simulink model "Simulasi_DIY"  (R2024b)
settings: Solver=VariableStepAuto  StartTime=0.0  StopTime=10.0  RelTol=1e-3
values from neighbouring files (symbols this model uses):
  d1 = l1/2    (= 0.5)    [parameter.m]
  d2 = l2/2    (= 0.5)    [parameter.m]
  g = 9.81    [parameter.m]
  I1 = 1/12*m1*l1^2    (= 0.0833333333333)    [parameter.m]
  I2 = 1/12*m2*l2^2    (= 0.0833333333333)    [parameter.m]
  Kpx = 400    [parameter.m]
  Kpy = 400    [parameter.m]
  Kvx = 150    [parameter.m]
  Kvy = 150    [parameter.m]
  l1 = 1    [parameter.m]
  l2 = 1    [parameter.m]
  m1 = 1    [parameter.m]
  m2 = 1    [parameter.m]
  xt = -1    [main.m]    (also in parameter.m)
  yt = 1    [main.m]    (also in parameter.m)
undefined symbols (not defined in the file or in its folder): the_init
settings Model: Creator=WIN 10  LastModifiedBy=rifki
settings RTWCC: GPUComputeCapability=3.5

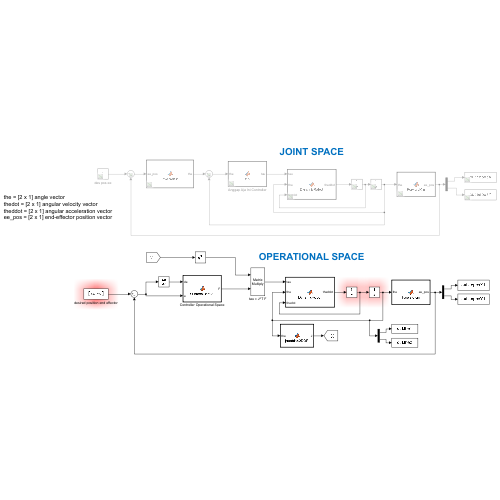
[thumbnail: Simulink's stored preview of the top-level diagram]
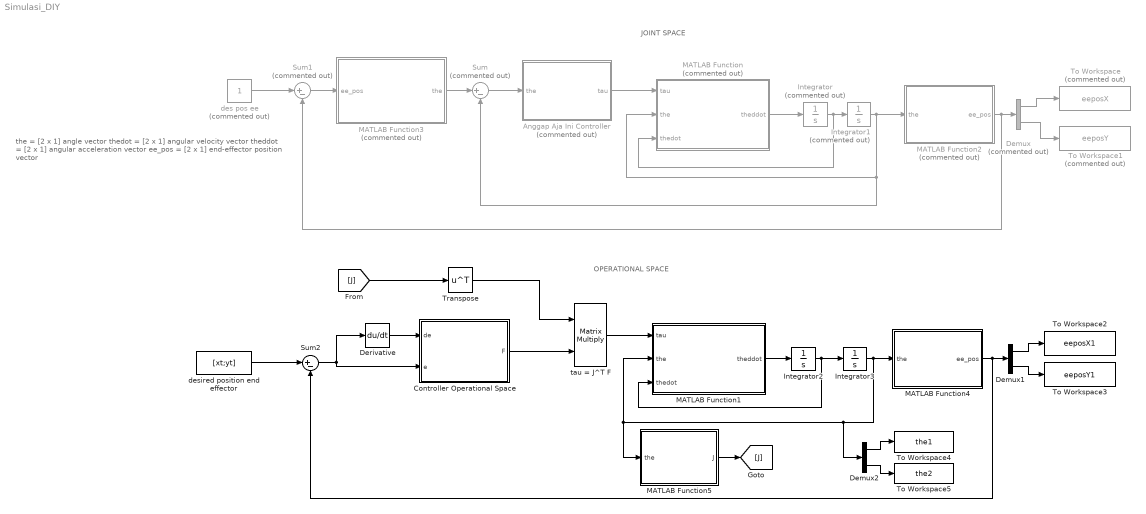
== system Simulasi_DIY ==
  note: JOINT SPACE
  note: the = [2 x 1] angle vector
      | thedot = [2 x 1] angular velocity vector
      | theddot = [2 x 1] angular acceleration vector
      | ee_pos = [2 x 1] end-effector position vector
  note: OPERATIONAL SPACE
  Anggap Aja Ini Controller : MATLAB Function  Commented=on  TreatAsAtomicUnit=on
  Controller Operational Space : MATLAB Function  TreatAsAtomicUnit=on
  Demux : Demux  Commented=on  Outputs=2
  Demux1 : Demux  Outputs=2
  Demux2 : Demux  Outputs=2
  Derivative : Derivative
  Integrator : Integrator  Commented=on  InitialCondition=[the_init(2);the_init(4)]
  Integrator1 : Integrator  Commented=on  InitialCondition=[the_init(1);the_init(3)]
  Integrator2 : Integrator  InitialCondition=[the_init(2);the_init(4)]
  Integrator3 : Integrator  InitialCondition=[the_init(1);the_init(3)]
  MATLAB Function : MATLAB Function  Commented=on  TreatAsAtomicUnit=on
  MATLAB Function1 : MATLAB Function  TreatAsAtomicUnit=on
  MATLAB Function2 : MATLAB Function  Commented=on  TreatAsAtomicUnit=on
  MATLAB Function3 : MATLAB Function  Commented=on  TreatAsAtomicUnit=on
  MATLAB Function4 : MATLAB Function  TreatAsAtomicUnit=on
  MATLAB Function5 : MATLAB Function  TreatAsAtomicUnit=on
  Sum : Sum  Commented=on  Inputs=|+-
  Sum1 : Sum  Commented=on  Inputs=|+-
  Sum2 : Sum  Inputs=|+-
  To Workspace : ToWorkspace  Commented=on  VariableName=eeposX  SaveFormat=Timeseries  SampleTime=-1
  To Workspace1 : ToWorkspace  Commented=on  VariableName=eeposY  SaveFormat=Timeseries  SampleTime=-1
  To Workspace2 : ToWorkspace  VariableName=eeposX1  SaveFormat=Timeseries  SampleTime=-1
  To Workspace3 : ToWorkspace  VariableName=eeposY1  SaveFormat=Timeseries  SampleTime=-1
  To Workspace4 : ToWorkspace  VariableName=the1  SaveFormat=Timeseries  SampleTime=-1
  To Workspace5 : ToWorkspace  VariableName=the2  SaveFormat=Timeseries  SampleTime=-1
  Transpose : Math  Operator=transpose
  des pos ee : Constant  Commented=on
  desired position end effector : Constant  Value=[xt;yt]
  tau = J^T F : Product  Multiplication=Matrix(*)
  wires:
  MATLAB Function/1(theddot) -> Integrator/1
  Integrator/1 -> MATLAB Function/3(thedot), Integrator1/1
  Integrator1/1 -> MATLAB Function/2(the), Sum/2, MATLAB Function2/1(the)
  Anggap Aja Ini Controller/1(tau) -> MATLAB Function/1(tau)
  Sum/1 -> Anggap Aja Ini Controller/1(the)
  MATLAB Function2/1(ee_pos) -> Sum1/2, Demux/1
  Demux/1 -> To Workspace/1
  Demux/2 -> To Workspace1/1
  MATLAB Function3/1(the) -> Sum/1
  Sum1/1 -> MATLAB Function3/1(ee_pos)
  MATLAB Function1/1(theddot) -> Integrator2/1
  Integrator2/1 -> MATLAB Function1/3(thedot), Integrator3/1
  Integrator3/1 -> Demux2/1, MATLAB Function1/2(the), MATLAB Function5/1(the), MATLAB Function4/1(the)
  Controller Operational Space/1(F) -> tau = J^T F/2
  tau = J^T F/1 -> MATLAB Function1/1(tau)
  Sum2/1 -> Derivative/1, Controller Operational Space/2(e)
  MATLAB Function4/1(ee_pos) -> Demux1/1, Sum2/2
  Demux1/1 -> To Workspace2/1
  Demux1/2 -> To Workspace3/1
  desired position end effector/1 -> Sum2/1
  des pos ee/1 -> Sum1/1
  MATLAB Function5/1(J) -> [J]
  Transpose/1 -> tau = J^T F/1
  [J] -> Transpose/1
  Derivative/1 -> Controller Operational Space/1(de)
  Demux2/1 -> To Workspace4/1
  Demux2/2 -> To Workspace5/1

== matlab function Simulasi_DIY/MATLAB Function5 ==
  data: the input; J output; l1 parameter; l2 parameter
function J = jacobian2DOF(the, l1, l2)
    % jacobian2DOF - Menghitung matriks Jacobian untuk robot 2DOF
    %
    % Sintaks:
    % J = jacobian2DOF(theta1, theta2, l1, l2)
    %
    % Input:
    % theta1 - Sudut sendi pertama (dalam radian)
    % theta2 - Sudut sendi kedua (dalam radian)
    % l1 - Panjang link pertama
    % l2 - Panjang link kedua
    %
    % Output:
    % J - Matriks Jacobian (2x2)

    the1 = the(1);
    the2 = the(2);
    
    % Elemen-elemen Jacobian
    J11 = -l1 * sin(the1) - l2 * sin(the1 + the2);
    J12 = -l2 * sin(the1 + the2);
    J21 = l1 * cos(the1) + l2 * cos(the1 + the2);
    J22 = l2 * cos(the1 + the2);
    
    % Matriks Jacobian
    J = [J11, J12; J21, J22];

== matlab function Simulasi_DIY/MATLAB Function ==
  data: tau input; l1 parameter; l2 parameter; d1 parameter; d2 parameter; m1 parameter; I1 parameter; I2 parameter; g parameter; the input; theddot output; thedot input
function theddot = DynamicRobot(tau,l1, l2, d1, d2, m1, I1, I2, g, the, thedot)

tau1 = tau(1);
tau2 = tau(2);

the1 = the(1);
the2 = the(2);

thedot1 = thedot(1);
thedot2 = thedot(2);

H11 = m1*d1^2 + I1 + m2*(l1^2 + d2^2 + 2*l1*l2*cos(the2)) + I2;
H22 = m2*d2^2 + I2;
H12 = m2*l1*d2*cos(the2) + m2*d2^2 + I2;
h = m2*l1*d2*sin(the2);
G1 = m1*d1*g*cos(the1) + m2*g*(l2*cos(the1+the2) + l1*cos(the1));
G2 = m2*d2*g*cos(the1+the2);

H = [H11 H12;H12 H22];
theddot = H\([tau1; tau2] - [-2*h*thedot2 -h*thedot2;h*thedot1 0]*[thedot1;thedot2] - [G1;G2]);

== matlab function Simulasi_DIY/MATLAB Function2 ==
  data: ee_pos output; the input; l1 parameter; l2 parameter
function ee_pos = ForwardKin(the, l1, l2)
%ForwardKin
%    RA_E = ForwardKin(L1,L2,TH1,TH2)

%    This function was generated by the Symbolic Math Toolbox version 9.3.
%    21-Jun-2024 03:34:29
the1 = the(1);
the2 = the(2);

t2 = the1+the2;
ee_pos = [l2.*cos(t2)+l1.*cos(the1); % x
    l2.*sin(t2)+l1.*sin(the1); % y
    0.0]; % z
end

== matlab function Simulasi_DIY/MATLAB Function3 ==
  data: ee_pos input; the output; l1 parameter; l2 parameter
function the = InverseKin(ee_pos, l1, l2)
    % inverseKinematics2DOF - Menghitung inverse kinematics untuk robot 2DOF
    % 
    % Sintaks:
    % [the1, the2] = inverseKinematics2DOF(x, y, l1, l2)
    % 
    % Input:
    % x - Koordinat x dari end-effector
    % y - Koordinat y dari end-effector
    % l1 - Panjang link pertama
    % l2 - Panjang link kedua
    %
    % Output:
    % the1 - Sudut sendi pertama (dalam radian)
    % the2 - Sudut sendi kedua (dalam radian)

    x = ee_pos(1);
    y = ee_pos(2);

    % Memastikan nilai input berada dalam jangkauan
    if sqrt(x^2 + y^2) > (l1 + l2)
        error('Posisi end-effector di luar jangkauan robot');
    end

    % Menghitung sudut sendi kedua
    cos_the2 = (x^2 + y^2 - l1^2 - l2^2) / (2 * l1 * l2);
    sin_the2 = sqrt(1 - cos_the2^2); % Memilih solusi elbow-up

    the2 = atan2(sin_the2, cos_the2);

    % Menghitung sudut sendi pertama
    k1 = l1 + l2 * cos(the2);
    k2 = l2 * sin(the2);
    the1 = atan2(y, x) - atan2(k2, k1);

    the = [the1, the2];
end

== matlab function Simulasi_DIY/Anggap Aja Ini Controller ==
  data: the input; tau output
function tau = fcn(the)

tau = the;

== matlab function Simulasi_DIY/MATLAB Function1 ==
  data: tau input; l1 parameter; l2 parameter; d1 parameter; d2 parameter; m1 parameter; I1 parameter; I2 parameter; g parameter; the input; theddot output; thedot input; m2 parameter
function theddot = DynamicRobot(tau,l1, l2, d1, d2, m1, I1, I2, g, the, thedot, m2)

tau1 = tau(1);
tau2 = tau(2);

the1 = the(1);
the2 = the(2);

thedot1 = thedot(1);
thedot2 = thedot(2);

H11 = m1*d1^2 + I1 + m2*(l1^2 + d2^2 + 2*l1*l2*cos(the2)) + I2;
H22 = m2*d2^2 + I2;
H12 = m2*l1*d2*cos(the2) + m2*d2^2 + I2;
h = m2*l1*d2*sin(the2);
G1 = m1*d1*g*cos(the1) + m2*g*(l2*cos(the1+the2) + l1*cos(the1));
G2 = m2*d2*g*cos(the1+the2);

H = [H11 H12;H12 H22];
theddot = H\([tau1; tau2] - [-2*h*thedot2 -h*thedot2;h*thedot1 0]*[thedot1;thedot2] - [G1;G2]);
% theddot = H\([tau1; tau2] - [-2*h*thedot2 -h*thedot2;h*thedot1
% 0]*[thedot1;thedot2]); % ignore gravity component

== matlab function Simulasi_DIY/MATLAB Function4 ==
  data: ee_pos output; the input; l1 parameter; l2 parameter
function ee_pos = ForwardKin(the, l1, l2)
%ForwardKin
%    RA_E = ForwardKin(L1,L2,TH1,TH2)

%    This function was generated by the Symbolic Math Toolbox version 9.3.
%    21-Jun-2024 03:34:29
the1 = the(1);
the2 = the(2);

t2 = the1+the2;
ee_pos = [l2.*cos(t2)+l1.*cos(the1); % x
    l2.*sin(t2)+l1.*sin(the1)]; % y
end

== matlab function Simulasi_DIY/Controller Operational Space ==
  data: de input; e input; Kpx parameter; F output; Kpy parameter; Kvx parameter; Kvy parameter
function F = StifnessControl(de,e,Kpx,Kpy, Kvx, Kvy)
ex = e(1);
ey = e(2);

dex = de(1);
dey = de(2);

Fx = Kpx*ex + Kvx*dex;
Fy = Kpy*ey + Kvy*dey;

F = [Fx;Fy];
